simulink model "TST_InjCrv_PoI2"  (R2016b)
settings: Solver=FixedStepDiscrete  StartTime=0.0  StopTime=simTime  FixedStep=sampleTime  RelTol=1e-3
values from neighbouring files (symbols this model uses):
  testCase = 1    [initTST_InjCrv_PoI2_001.m]    (also in initTST_InjCrv_PoI2_002.m = 2)
libraries: simulink x6
settings Model: Creator=WF305  LastModifiedBy=WF305
settings DebuggingCC: SignalRangeChecking=error

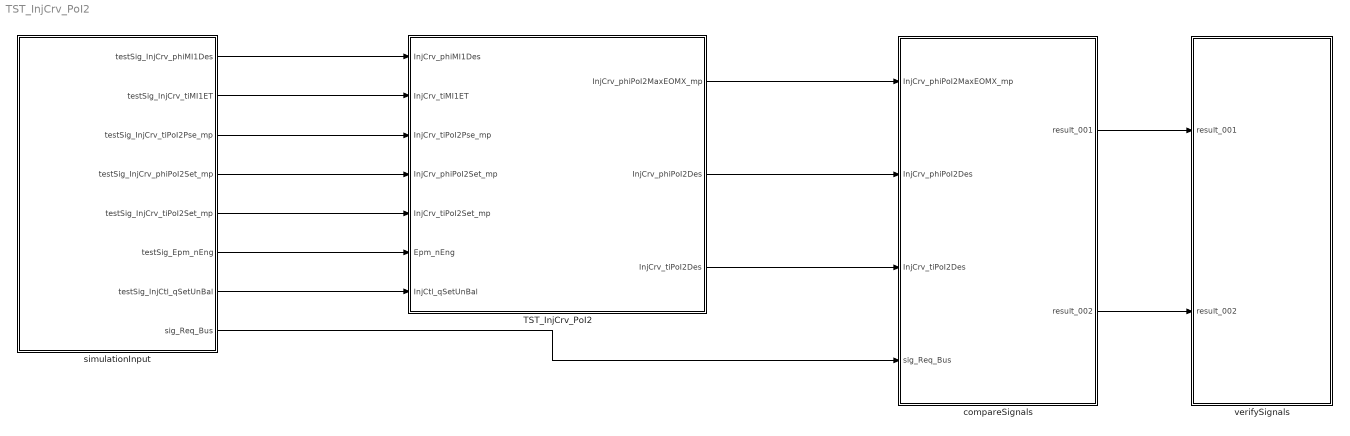
== system TST_InjCrv_PoI2 ==
  TST_InjCrv_PoI2 : Subsystem
  compareSignals : Subsystem
  simulationInput : Subsystem
  verifySignals : Subsystem
  wires:
  simulationInput/1(testSig_InjCrv_phiMI1Des) -> TST_InjCrv_PoI2/1(InjCrv_phiMI1Des)
  simulationInput/2(testSig_InjCrv_tiMI1ET) -> TST_InjCrv_PoI2/2(InjCrv_tiMI1ET)
  simulationInput/3(testSig_InjCrv_tiPoI2Pse_mp) -> TST_InjCrv_PoI2/3(InjCrv_tiPoI2Pse_mp)
  simulationInput/4(testSig_InjCrv_phiPoI2Set_mp) -> TST_InjCrv_PoI2/4(InjCrv_phiPoI2Set_mp)
  simulationInput/5(testSig_InjCrv_tiPoI2Set_mp) -> TST_InjCrv_PoI2/5(InjCrv_tiPoI2Set_mp)
  simulationInput/6(testSig_Epm_nEng) -> TST_InjCrv_PoI2/6(Epm_nEng)
  simulationInput/7(testSig_InjCtl_qSetUnBal) -> TST_InjCrv_PoI2/7(InjCtl_qSetUnBal)
  TST_InjCrv_PoI2/1(InjCrv_phiPoI2MaxEOMX_mp) -> compareSignals/1(InjCrv_phiPoI2MaxEOMX_mp)
  TST_InjCrv_PoI2/2(InjCrv_phiPoI2Des) -> compareSignals/2(InjCrv_phiPoI2Des)
  TST_InjCrv_PoI2/3(InjCrv_tiPoI2Des) -> compareSignals/3(InjCrv_tiPoI2Des)
  simulationInput/8(sig_Req_Bus) -> compareSignals/4(sig_Req_Bus)
  compareSignals/1(result_001) -> verifySignals/1(result_001)
  compareSignals/2(result_002) -> verifySignals/2(result_002)

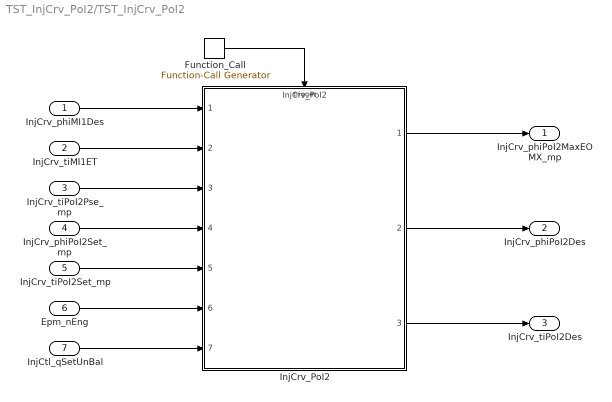
== system TST_InjCrv_PoI2/TST_InjCrv_PoI2 ==
  InjCrv_phiMI1Des : Inport
  InjCrv_tiMI1ET : Inport  Port=2
  InjCrv_tiPoI2Pse_mp : Inport  Port=3
  InjCrv_phiPoI2Set_mp : Inport  Port=4
  InjCrv_tiPoI2Set_mp : Inport  Port=5
  Epm_nEng : Inport  Port=6
  InjCtl_qSetUnBal : Inport  Port=7
  Function_Call : simulink/Ports & Subsystems/Function-Call Generator  sample_time=sampleTime  numberOfIterations=1
  InjCrv_PoI2 : ModelReference  ModelNameDialog=InjCrv_PoI2  ModelReferenceVersion=1.22  TriggerPortName=function  TriggerPortTriggerType=function-call  TriggerPortStatesWhenEnabling=held
  InjCrv_phiPoI2MaxEOMX_mp : Outport
  InjCrv_phiPoI2Des : Outport  Port=2
  InjCrv_tiPoI2Des : Outport  Port=3
  wires:
  Function_Call/1 -> InjCrv_PoI2/Trigger
  InjCrv_phiMI1Des/1 -> InjCrv_PoI2/1
  InjCrv_tiMI1ET/1 -> InjCrv_PoI2/2
  InjCrv_tiPoI2Pse_mp/1 -> InjCrv_PoI2/3
  InjCrv_phiPoI2Set_mp/1 -> InjCrv_PoI2/4
  InjCrv_tiPoI2Set_mp/1 -> InjCrv_PoI2/5
  Epm_nEng/1 -> InjCrv_PoI2/6
  InjCtl_qSetUnBal/1 -> InjCrv_PoI2/7
  InjCrv_PoI2/1 -> InjCrv_phiPoI2MaxEOMX_mp/1
  InjCrv_PoI2/2 -> InjCrv_phiPoI2Des/1
  InjCrv_PoI2/3 -> InjCrv_tiPoI2Des/1

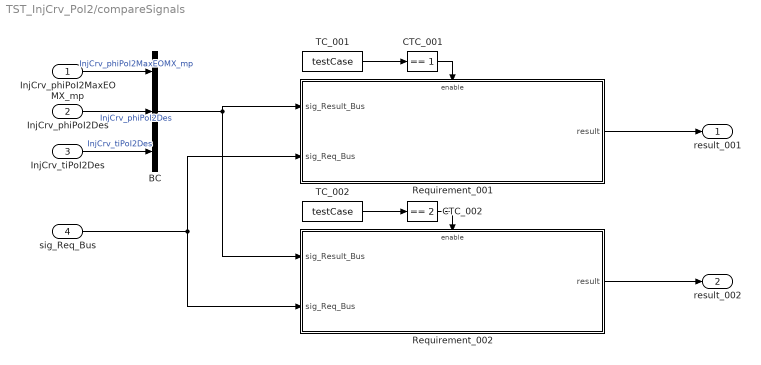
== system TST_InjCrv_PoI2/compareSignals ==
  InjCrv_phiPoI2MaxEOMX_mp : Inport
  InjCrv_phiPoI2Des : Inport  Port=2
  InjCrv_tiPoI2Des : Inport  Port=3
  sig_Req_Bus : Inport  Port=4
  BC : BusCreator  Inputs=3
  CTC_001 : simulink/Logic and Bit Operations/Compare To Constant  relop===  const=1  OutDataTypeStr=boolean
  CTC_002 : simulink/Logic and Bit Operations/Compare To Constant  relop===  const=2  OutDataTypeStr=boolean
  Requirement_001 : Subsystem
  Requirement_002 : Subsystem
  TC_001 : Constant  Value=testCase
  TC_002 : Constant  Value=testCase
  result_001 : Outport
  result_002 : Outport  Port=2
  wires:
  InjCrv_phiPoI2MaxEOMX_mp/1 -> BC/1  "InjCrv_phiPoI2MaxEOMX_mp"
  InjCrv_phiPoI2Des/1 -> BC/2  "InjCrv_phiPoI2Des"
  InjCrv_tiPoI2Des/1 -> BC/3  "InjCrv_tiPoI2Des"
  TC_001/1 -> CTC_001/1
  CTC_001/1 -> Requirement_001/Enable
  sig_Req_Bus/1 -> Requirement_001/2(sig_Req_Bus), Requirement_002/2(sig_Req_Bus)
  BC/1 -> Requirement_001/1(sig_Result_Bus), Requirement_002/1(sig_Result_Bus)
  Requirement_001/1(result) -> result_001/1
  TC_002/1 -> CTC_002/1
  CTC_002/1 -> Requirement_002/Enable
  Requirement_002/1(result) -> result_002/1

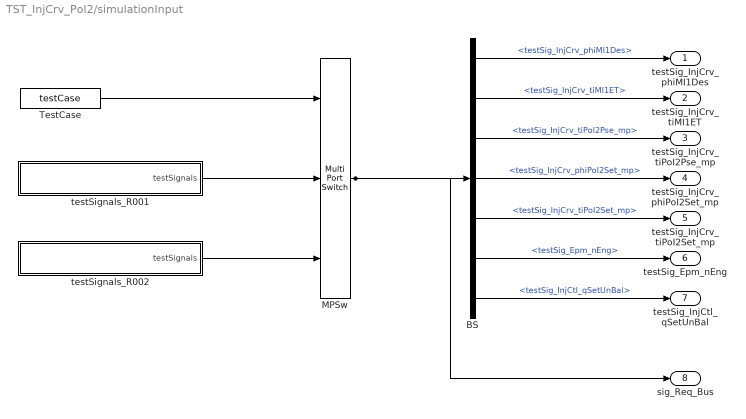
== system TST_InjCrv_PoI2/simulationInput ==
  BS : BusSelector  OutputSignals=testSig_InjCrv_phiMI1Des,testSig_InjCrv_tiMI1ET,testSig_InjCrv_tiPoI2Pse_mp,testSig_InjCrv_phiPoI2Set_mp,testSig_InjCrv_tiPoI2Set_mp,testSig_Epm_nEng,testSig_InjCtl_qSetUnBal
  MPSw : MultiPortSwitch  Inputs=2  SaturateOnIntegerOverflow=on  InputSameDT=on
  TestCase : Constant  Value=testCase
  testSignals_R001 : Subsystem
  testSignals_R002 : Subsystem
  testSig_InjCrv_phiMI1Des : Outport
  testSig_InjCrv_tiMI1ET : Outport  Port=2
  testSig_InjCrv_tiPoI2Pse_mp : Outport  Port=3
  testSig_InjCrv_phiPoI2Set_mp : Outport  Port=4
  testSig_InjCrv_tiPoI2Set_mp : Outport  Port=5
  testSig_Epm_nEng : Outport  Port=6
  testSig_InjCtl_qSetUnBal : Outport  Port=7
  sig_Req_Bus : Outport  Port=8
  wires:
  BS/1 -> testSig_InjCrv_phiMI1Des/1  "<testSig_InjCrv_phiMI1Des>"
  BS/2 -> testSig_InjCrv_tiMI1ET/1  "<testSig_InjCrv_tiMI1ET>"
  BS/3 -> testSig_InjCrv_tiPoI2Pse_mp/1  "<testSig_InjCrv_tiPoI2Pse_mp>"
  BS/4 -> testSig_InjCrv_phiPoI2Set_mp/1  "<testSig_InjCrv_phiPoI2Set_mp>"
  BS/5 -> testSig_InjCrv_tiPoI2Set_mp/1  "<testSig_InjCrv_tiPoI2Set_mp>"
  BS/6 -> testSig_Epm_nEng/1  "<testSig_Epm_nEng>"
  BS/7 -> testSig_InjCtl_qSetUnBal/1  "<testSig_InjCtl_qSetUnBal>"
  MPSw/1 -> BS/1, sig_Req_Bus/1
  TestCase/1 -> MPSw/1
  testSignals_R001/1(testSignals) -> MPSw/2
  testSignals_R002/1(testSignals) -> MPSw/3

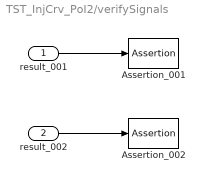
== system TST_InjCrv_PoI2/verifySignals ==
  result_001 : Inport
  result_002 : Inport  Port=2
  Assertion_001 : Assertion  Enabled=off
  Assertion_002 : Assertion  Enabled=off
  wires:
  result_001/1 -> Assertion_001/1
  result_002/1 -> Assertion_002/1

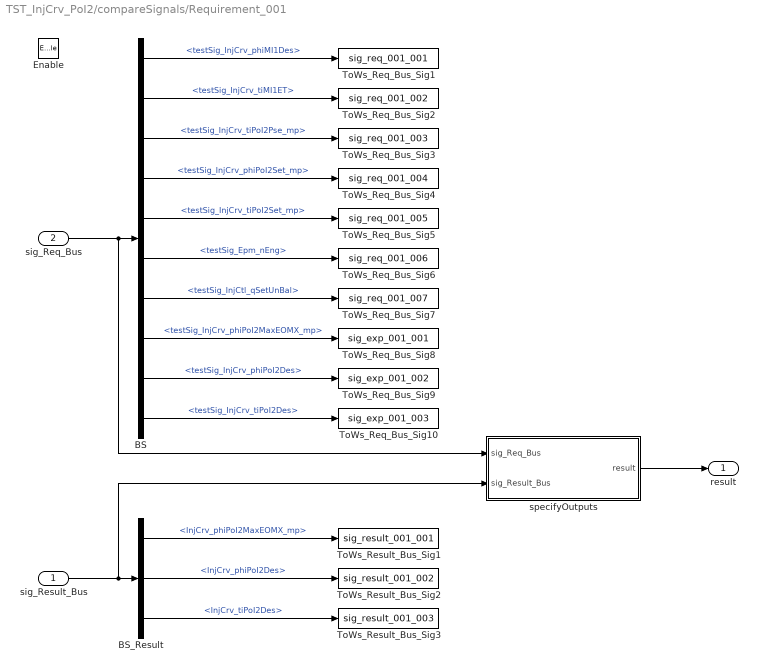
== system TST_InjCrv_PoI2/compareSignals/Requirement_001 ==
  sig_Result_Bus : Inport
  sig_Req_Bus : Inport  Port=2
  Enable : EnablePort
  BS : BusSelector  OutputSignals=testSig_InjCrv_phiMI1Des,testSig_InjCrv_tiMI1ET,testSig_InjCrv_tiPoI2Pse_mp,testSig_InjCrv_phiPoI2Set_mp,testSig_InjCrv_tiPoI2Set_mp,testSig_Epm_nEng,testSig_InjCtl_qSetUnBal,testSig_InjCrv_phiPoI2MaxEOMX_mp,testSig_InjCrv_phiPoI2Des,testSig_InjCrv_tiPoI2Des
  BS_Result : BusSelector  OutputSignals=InjCrv_phiPoI2MaxEOMX_mp,InjCrv_phiPoI2Des,InjCrv_tiPoI2Des
  ToWs_Req_Bus_Sig1 : ToWorkspace  VariableName=sig_req_001_001  SaveFormat=Structure With Time
  ToWs_Req_Bus_Sig10 : ToWorkspace  VariableName=sig_exp_001_003  SaveFormat=Structure With Time
  ToWs_Req_Bus_Sig2 : ToWorkspace  VariableName=sig_req_001_002  SaveFormat=Structure With Time
  ToWs_Req_Bus_Sig3 : ToWorkspace  VariableName=sig_req_001_003  SaveFormat=Structure With Time
  ToWs_Req_Bus_Sig4 : ToWorkspace  VariableName=sig_req_001_004  SaveFormat=Structure With Time
  ToWs_Req_Bus_Sig5 : ToWorkspace  VariableName=sig_req_001_005  SaveFormat=Structure With Time
  ToWs_Req_Bus_Sig6 : ToWorkspace  VariableName=sig_req_001_006  SaveFormat=Structure With Time
  ToWs_Req_Bus_Sig7 : ToWorkspace  VariableName=sig_req_001_007  SaveFormat=Structure With Time
  ToWs_Req_Bus_Sig8 : ToWorkspace  VariableName=sig_exp_001_001  SaveFormat=Structure With Time
  ToWs_Req_Bus_Sig9 : ToWorkspace  VariableName=sig_exp_001_002  SaveFormat=Structure With Time
  ToWs_Result_Bus_Sig1 : ToWorkspace  VariableName=sig_result_001_001  SaveFormat=Structure With Time
  ToWs_Result_Bus_Sig2 : ToWorkspace  VariableName=sig_result_001_002  SaveFormat=Structure With Time
  ToWs_Result_Bus_Sig3 : ToWorkspace  VariableName=sig_result_001_003  SaveFormat=Structure With Time
  specifyOutputs : Subsystem
  result : Outport
  wires:
  sig_Req_Bus/1 -> BS/1, specifyOutputs/1(sig_Req_Bus)
  BS/1 -> ToWs_Req_Bus_Sig1/1  "<testSig_InjCrv_phiMI1Des>"
  BS/2 -> ToWs_Req_Bus_Sig2/1  "<testSig_InjCrv_tiMI1ET>"
  BS/3 -> ToWs_Req_Bus_Sig3/1  "<testSig_InjCrv_tiPoI2Pse_mp>"
  BS/4 -> ToWs_Req_Bus_Sig4/1  "<testSig_InjCrv_phiPoI2Set_mp>"
  BS/5 -> ToWs_Req_Bus_Sig5/1  "<testSig_InjCrv_tiPoI2Set_mp>"
  BS/6 -> ToWs_Req_Bus_Sig6/1  "<testSig_Epm_nEng>"
  BS/7 -> ToWs_Req_Bus_Sig7/1  "<testSig_InjCtl_qSetUnBal>"
  BS/8 -> ToWs_Req_Bus_Sig8/1  "<testSig_InjCrv_phiPoI2MaxEOMX_mp>"
  BS/9 -> ToWs_Req_Bus_Sig9/1  "<testSig_InjCrv_phiPoI2Des>"
  BS/10 -> ToWs_Req_Bus_Sig10/1  "<testSig_InjCrv_tiPoI2Des>"
  sig_Result_Bus/1 -> BS_Result/1, specifyOutputs/2(sig_Result_Bus)
  BS_Result/1 -> ToWs_Result_Bus_Sig1/1  "<InjCrv_phiPoI2MaxEOMX_mp>"
  BS_Result/2 -> ToWs_Result_Bus_Sig2/1  "<InjCrv_phiPoI2Des>"
  BS_Result/3 -> ToWs_Result_Bus_Sig3/1  "<InjCrv_tiPoI2Des>"
  specifyOutputs/1(result) -> result/1

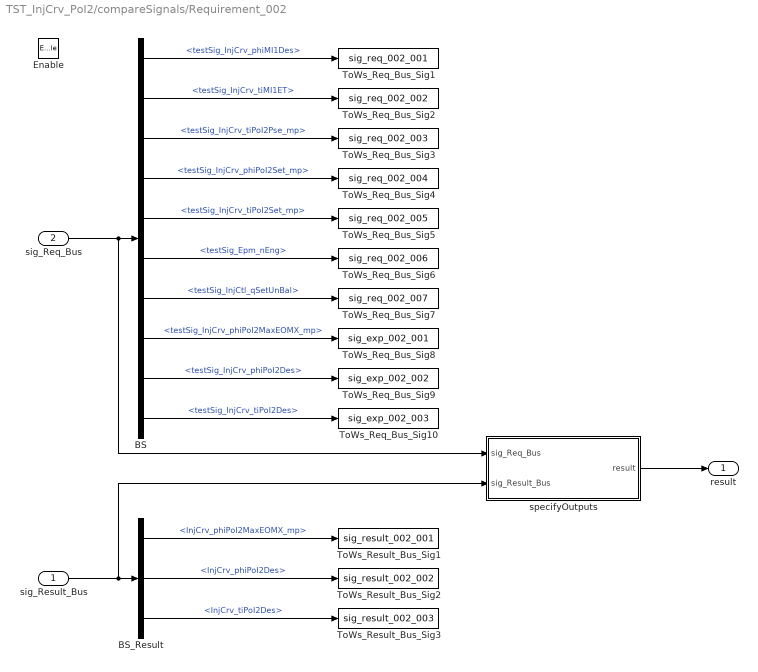
== system TST_InjCrv_PoI2/compareSignals/Requirement_002 ==
  sig_Result_Bus : Inport
  sig_Req_Bus : Inport  Port=2
  Enable : EnablePort
  BS : BusSelector  OutputSignals=testSig_InjCrv_phiMI1Des,testSig_InjCrv_tiMI1ET,testSig_InjCrv_tiPoI2Pse_mp,testSig_InjCrv_phiPoI2Set_mp,testSig_InjCrv_tiPoI2Set_mp,testSig_Epm_nEng,testSig_InjCtl_qSetUnBal,testSig_InjCrv_phiPoI2MaxEOMX_mp,testSig_InjCrv_phiPoI2Des,testSig_InjCrv_tiPoI2Des
  BS_Result : BusSelector  OutputSignals=InjCrv_phiPoI2MaxEOMX_mp,InjCrv_phiPoI2Des,InjCrv_tiPoI2Des
  ToWs_Req_Bus_Sig1 : ToWorkspace  VariableName=sig_req_002_001  SaveFormat=Structure With Time
  ToWs_Req_Bus_Sig10 : ToWorkspace  VariableName=sig_exp_002_003  SaveFormat=Structure With Time
  ToWs_Req_Bus_Sig2 : ToWorkspace  VariableName=sig_req_002_002  SaveFormat=Structure With Time
  ToWs_Req_Bus_Sig3 : ToWorkspace  VariableName=sig_req_002_003  SaveFormat=Structure With Time
  ToWs_Req_Bus_Sig4 : ToWorkspace  VariableName=sig_req_002_004  SaveFormat=Structure With Time
  ToWs_Req_Bus_Sig5 : ToWorkspace  VariableName=sig_req_002_005  SaveFormat=Structure With Time
  ToWs_Req_Bus_Sig6 : ToWorkspace  VariableName=sig_req_002_006  SaveFormat=Structure With Time
  ToWs_Req_Bus_Sig7 : ToWorkspace  VariableName=sig_req_002_007  SaveFormat=Structure With Time
  ToWs_Req_Bus_Sig8 : ToWorkspace  VariableName=sig_exp_002_001  SaveFormat=Structure With Time
  ToWs_Req_Bus_Sig9 : ToWorkspace  VariableName=sig_exp_002_002  SaveFormat=Structure With Time
  ToWs_Result_Bus_Sig1 : ToWorkspace  VariableName=sig_result_002_001  SaveFormat=Structure With Time
  ToWs_Result_Bus_Sig2 : ToWorkspace  VariableName=sig_result_002_002  SaveFormat=Structure With Time
  ToWs_Result_Bus_Sig3 : ToWorkspace  VariableName=sig_result_002_003  SaveFormat=Structure With Time
  specifyOutputs : Subsystem
  result : Outport
  wires:
  sig_Req_Bus/1 -> BS/1, specifyOutputs/1(sig_Req_Bus)
  BS/1 -> ToWs_Req_Bus_Sig1/1  "<testSig_InjCrv_phiMI1Des>"
  BS/2 -> ToWs_Req_Bus_Sig2/1  "<testSig_InjCrv_tiMI1ET>"
  BS/3 -> ToWs_Req_Bus_Sig3/1  "<testSig_InjCrv_tiPoI2Pse_mp>"
  BS/4 -> ToWs_Req_Bus_Sig4/1  "<testSig_InjCrv_phiPoI2Set_mp>"
  BS/5 -> ToWs_Req_Bus_Sig5/1  "<testSig_InjCrv_tiPoI2Set_mp>"
  BS/6 -> ToWs_Req_Bus_Sig6/1  "<testSig_Epm_nEng>"
  BS/7 -> ToWs_Req_Bus_Sig7/1  "<testSig_InjCtl_qSetUnBal>"
  BS/8 -> ToWs_Req_Bus_Sig8/1  "<testSig_InjCrv_phiPoI2MaxEOMX_mp>"
  BS/9 -> ToWs_Req_Bus_Sig9/1  "<testSig_InjCrv_phiPoI2Des>"
  BS/10 -> ToWs_Req_Bus_Sig10/1  "<testSig_InjCrv_tiPoI2Des>"
  sig_Result_Bus/1 -> BS_Result/1, specifyOutputs/2(sig_Result_Bus)
  BS_Result/1 -> ToWs_Result_Bus_Sig1/1  "<InjCrv_phiPoI2MaxEOMX_mp>"
  BS_Result/2 -> ToWs_Result_Bus_Sig2/1  "<InjCrv_phiPoI2Des>"
  BS_Result/3 -> ToWs_Result_Bus_Sig3/1  "<InjCrv_tiPoI2Des>"
  specifyOutputs/1(result) -> result/1

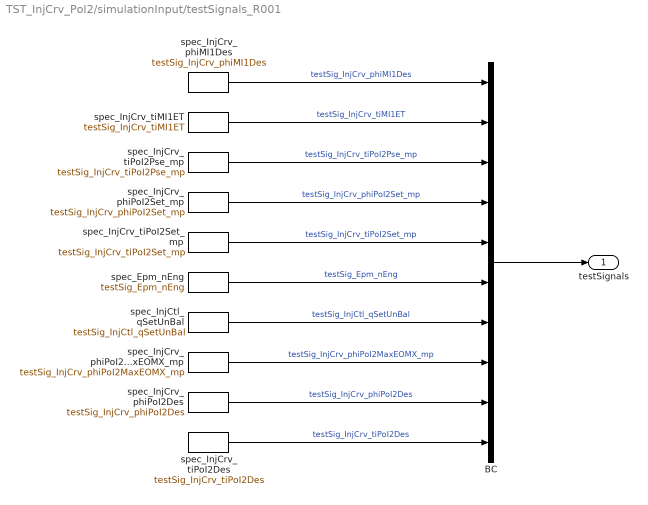
== system TST_InjCrv_PoI2/simulationInput/testSignals_R001 ==
  BC : BusCreator  Inputs=10
  spec_Epm_nEng : FromWorkspace  VariableName=testSig_Epm_nEng  Interpolate=off  OutputAfterFinalValue=Holding final value
  spec_InjCrv_phiMI1Des : FromWorkspace  VariableName=testSig_InjCrv_phiMI1Des  Interpolate=off  OutputAfterFinalValue=Holding final value
  spec_InjCrv_phiPoI2Des : FromWorkspace  VariableName=testSig_InjCrv_phiPoI2Des  Interpolate=off  OutputAfterFinalValue=Holding final value
  spec_InjCrv_phiPoI2MaxEOMX_mp : FromWorkspace  VariableName=testSig_InjCrv_phiPoI2MaxEOMX_mp  Interpolate=off  OutputAfterFinalValue=Holding final value
  spec_InjCrv_phiPoI2Set_mp : FromWorkspace  VariableName=testSig_InjCrv_phiPoI2Set_mp  Interpolate=off  OutputAfterFinalValue=Holding final value
  spec_InjCrv_tiMI1ET : FromWorkspace  VariableName=testSig_InjCrv_tiMI1ET  Interpolate=off  OutputAfterFinalValue=Holding final value
  spec_InjCrv_tiPoI2Des : FromWorkspace  VariableName=testSig_InjCrv_tiPoI2Des  Interpolate=off  OutputAfterFinalValue=Holding final value
  spec_InjCrv_tiPoI2Pse_mp : FromWorkspace  VariableName=testSig_InjCrv_tiPoI2Pse_mp  Interpolate=off  OutputAfterFinalValue=Holding final value
  spec_InjCrv_tiPoI2Set_mp : FromWorkspace  VariableName=testSig_InjCrv_tiPoI2Set_mp  Interpolate=off  OutputAfterFinalValue=Holding final value
  spec_InjCtl_qSetUnBal : FromWorkspace  VariableName=testSig_InjCtl_qSetUnBal  Interpolate=off  OutputAfterFinalValue=Holding final value
  testSignals : Outport
  wires:
  BC/1 -> testSignals/1
  spec_InjCrv_phiMI1Des/1 -> BC/1  "testSig_InjCrv_phiMI1Des"
  spec_InjCrv_tiMI1ET/1 -> BC/2  "testSig_InjCrv_tiMI1ET"
  spec_InjCrv_tiPoI2Pse_mp/1 -> BC/3  "testSig_InjCrv_tiPoI2Pse_mp"
  spec_InjCrv_phiPoI2Set_mp/1 -> BC/4  "testSig_InjCrv_phiPoI2Set_mp"
  spec_InjCrv_tiPoI2Set_mp/1 -> BC/5  "testSig_InjCrv_tiPoI2Set_mp"
  spec_Epm_nEng/1 -> BC/6  "testSig_Epm_nEng"
  spec_InjCtl_qSetUnBal/1 -> BC/7  "testSig_InjCtl_qSetUnBal"
  spec_InjCrv_phiPoI2MaxEOMX_mp/1 -> BC/8  "testSig_InjCrv_phiPoI2MaxEOMX_mp"
  spec_InjCrv_phiPoI2Des/1 -> BC/9  "testSig_InjCrv_phiPoI2Des"
  spec_InjCrv_tiPoI2Des/1 -> BC/10  "testSig_InjCrv_tiPoI2Des"

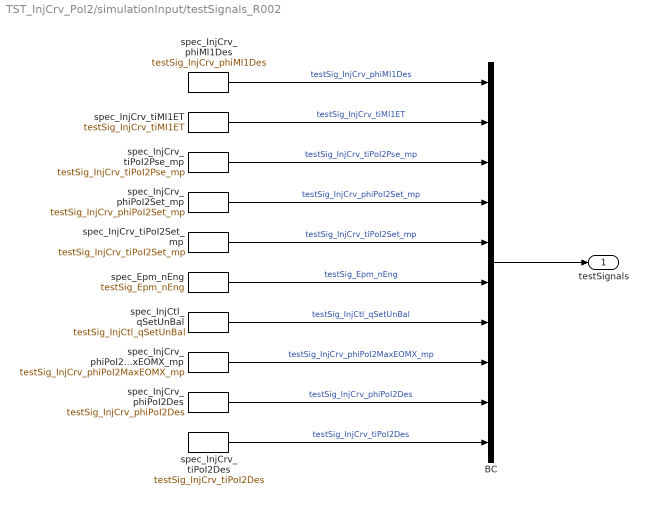
== system TST_InjCrv_PoI2/simulationInput/testSignals_R002 ==
  BC : BusCreator  Inputs=10
  spec_Epm_nEng : FromWorkspace  VariableName=testSig_Epm_nEng  Interpolate=off  OutputAfterFinalValue=Holding final value
  spec_InjCrv_phiMI1Des : FromWorkspace  VariableName=testSig_InjCrv_phiMI1Des  Interpolate=off  OutputAfterFinalValue=Holding final value
  spec_InjCrv_phiPoI2Des : FromWorkspace  VariableName=testSig_InjCrv_phiPoI2Des  Interpolate=off  OutputAfterFinalValue=Holding final value
  spec_InjCrv_phiPoI2MaxEOMX_mp : FromWorkspace  VariableName=testSig_InjCrv_phiPoI2MaxEOMX_mp  Interpolate=off  OutputAfterFinalValue=Holding final value
  spec_InjCrv_phiPoI2Set_mp : FromWorkspace  VariableName=testSig_InjCrv_phiPoI2Set_mp  Interpolate=off  OutputAfterFinalValue=Holding final value
  spec_InjCrv_tiMI1ET : FromWorkspace  VariableName=testSig_InjCrv_tiMI1ET  Interpolate=off  OutputAfterFinalValue=Holding final value
  spec_InjCrv_tiPoI2Des : FromWorkspace  VariableName=testSig_InjCrv_tiPoI2Des  Interpolate=off  OutputAfterFinalValue=Holding final value
  spec_InjCrv_tiPoI2Pse_mp : FromWorkspace  VariableName=testSig_InjCrv_tiPoI2Pse_mp  Interpolate=off  OutputAfterFinalValue=Holding final value
  spec_InjCrv_tiPoI2Set_mp : FromWorkspace  VariableName=testSig_InjCrv_tiPoI2Set_mp  Interpolate=off  OutputAfterFinalValue=Holding final value
  spec_InjCtl_qSetUnBal : FromWorkspace  VariableName=testSig_InjCtl_qSetUnBal  Interpolate=off  OutputAfterFinalValue=Holding final value
  testSignals : Outport
  wires:
  BC/1 -> testSignals/1
  spec_InjCrv_phiMI1Des/1 -> BC/1  "testSig_InjCrv_phiMI1Des"
  spec_InjCrv_tiMI1ET/1 -> BC/2  "testSig_InjCrv_tiMI1ET"
  spec_InjCrv_tiPoI2Pse_mp/1 -> BC/3  "testSig_InjCrv_tiPoI2Pse_mp"
  spec_InjCrv_phiPoI2Set_mp/1 -> BC/4  "testSig_InjCrv_phiPoI2Set_mp"
  spec_InjCrv_tiPoI2Set_mp/1 -> BC/5  "testSig_InjCrv_tiPoI2Set_mp"
  spec_Epm_nEng/1 -> BC/6  "testSig_Epm_nEng"
  spec_InjCtl_qSetUnBal/1 -> BC/7  "testSig_InjCtl_qSetUnBal"
  spec_InjCrv_phiPoI2MaxEOMX_mp/1 -> BC/8  "testSig_InjCrv_phiPoI2MaxEOMX_mp"
  spec_InjCrv_phiPoI2Des/1 -> BC/9  "testSig_InjCrv_phiPoI2Des"
  spec_InjCrv_tiPoI2Des/1 -> BC/10  "testSig_InjCrv_tiPoI2Des"

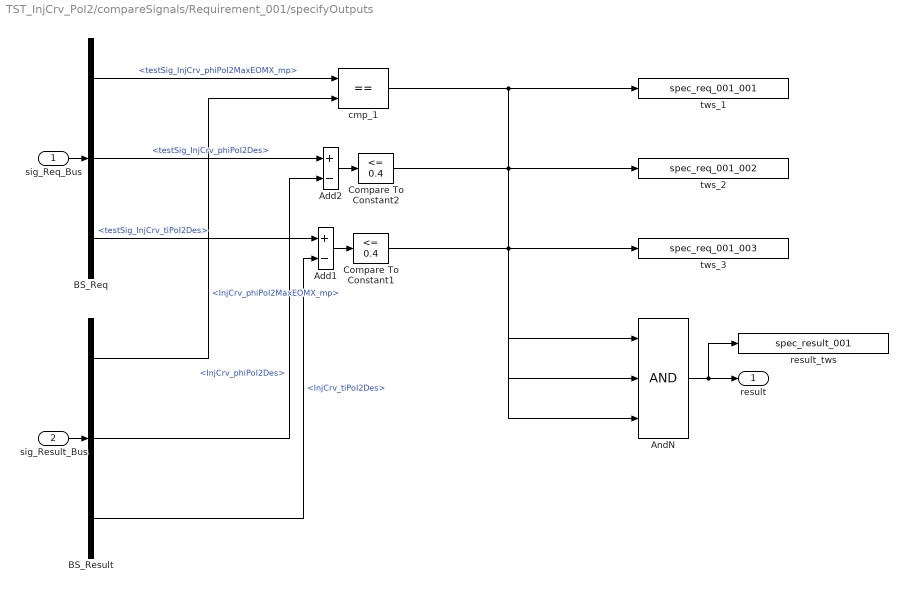
== system TST_InjCrv_PoI2/compareSignals/Requirement_001/specifyOutputs ==
  sig_Req_Bus : Inport
  sig_Result_Bus : Inport  Port=2
  Add1 : Sum  Inputs=+-
  Add2 : Sum  Inputs=+-
  AndN : Logic  Inputs=3
  BS_Req : BusSelector  OutputSignals=testSig_InjCrv_phiPoI2MaxEOMX_mp,testSig_InjCrv_phiPoI2Des,testSig_InjCrv_tiPoI2Des
  BS_Result : BusSelector  OutputSignals=InjCrv_phiPoI2MaxEOMX_mp,InjCrv_phiPoI2Des,InjCrv_tiPoI2Des
  Compare To Constant1 : simulink/Logic and Bit Operations/Compare To Constant  relop=<=  const=0.4  OutDataTypeStr=boolean
  Compare To Constant2 : simulink/Logic and Bit Operations/Compare To Constant  relop=<=  const=0.4  OutDataTypeStr=boolean
  cmp_1 : RelationalOperator  Operator===  RndMeth=Nearest  InputSameDT=on
  result_tws : ToWorkspace  VariableName=spec_result_001
  tws_1 : ToWorkspace  VariableName=spec_req_001_001
  tws_2 : ToWorkspace  VariableName=spec_req_001_002
  tws_3 : ToWorkspace  VariableName=spec_req_001_003
  result : Outport
  wires:
  sig_Req_Bus/1 -> BS_Req/1
  sig_Result_Bus/1 -> BS_Result/1
  AndN/1 -> result/1, result_tws/1
  BS_Req/1 -> cmp_1/1  "<testSig_InjCrv_phiPoI2MaxEOMX_mp>"
  BS_Result/1 -> cmp_1/2  "<InjCrv_phiPoI2MaxEOMX_mp>"
  cmp_1/1 -> tws_1/1, AndN/1
  BS_Req/2 -> Add2/1  "<testSig_InjCrv_phiPoI2Des>"
  BS_Result/2 -> Add2/2  "<InjCrv_phiPoI2Des>"
  Compare To Constant2/1 -> tws_2/1, AndN/2
  BS_Req/3 -> Add1/1  "<testSig_InjCrv_tiPoI2Des>"
  BS_Result/3 -> Add1/2  "<InjCrv_tiPoI2Des>"
  Compare To Constant1/1 -> tws_3/1, AndN/3
  Add1/1 -> Compare To Constant1/1
  Add2/1 -> Compare To Constant2/1

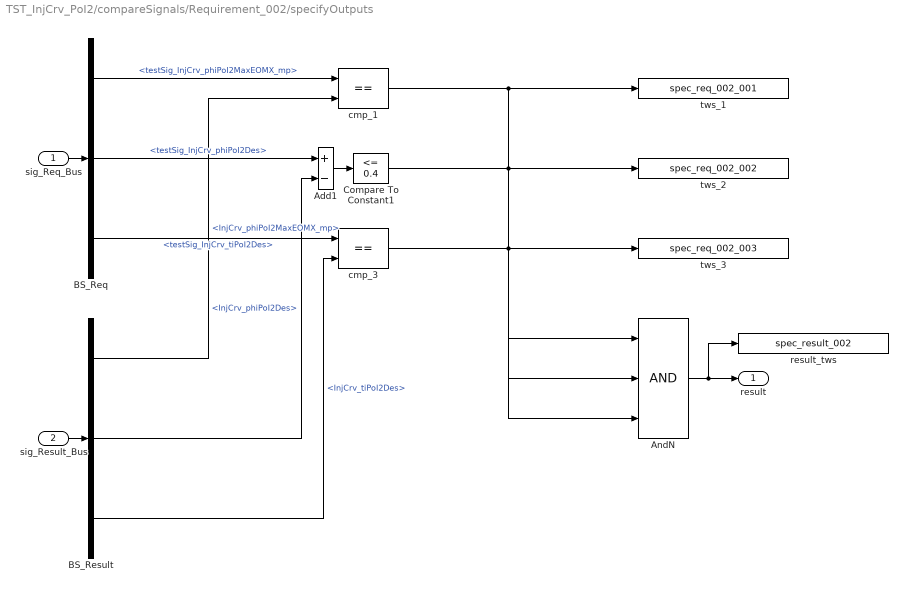
== system TST_InjCrv_PoI2/compareSignals/Requirement_002/specifyOutputs ==
  sig_Req_Bus : Inport
  sig_Result_Bus : Inport  Port=2
  Add1 : Sum  Inputs=+-
  AndN : Logic  Inputs=3
  BS_Req : BusSelector  OutputSignals=testSig_InjCrv_phiPoI2MaxEOMX_mp,testSig_InjCrv_phiPoI2Des,testSig_InjCrv_tiPoI2Des
  BS_Result : BusSelector  OutputSignals=InjCrv_phiPoI2MaxEOMX_mp,InjCrv_phiPoI2Des,InjCrv_tiPoI2Des
  Compare To Constant1 : simulink/Logic and Bit Operations/Compare To Constant  relop=<=  const=0.4  OutDataTypeStr=boolean
  cmp_1 : RelationalOperator  Operator===  RndMeth=Nearest  InputSameDT=on
  cmp_3 : RelationalOperator  Operator===  RndMeth=Nearest  InputSameDT=on
  result_tws : ToWorkspace  VariableName=spec_result_002
  tws_1 : ToWorkspace  VariableName=spec_req_002_001
  tws_2 : ToWorkspace  VariableName=spec_req_002_002
  tws_3 : ToWorkspace  VariableName=spec_req_002_003
  result : Outport
  wires:
  sig_Req_Bus/1 -> BS_Req/1
  sig_Result_Bus/1 -> BS_Result/1
  AndN/1 -> result/1, result_tws/1
  BS_Req/1 -> cmp_1/1  "<testSig_InjCrv_phiPoI2MaxEOMX_mp>"
  BS_Result/1 -> cmp_1/2  "<InjCrv_phiPoI2MaxEOMX_mp>"
  cmp_1/1 -> tws_1/1, AndN/1
  BS_Req/2 -> Add1/1  "<testSig_InjCrv_phiPoI2Des>"
  BS_Result/2 -> Add1/2  "<InjCrv_phiPoI2Des>"
  Compare To Constant1/1 -> tws_2/1, AndN/2
  BS_Req/3 -> cmp_3/1  "<testSig_InjCrv_tiPoI2Des>"
  BS_Result/3 -> cmp_3/2  "<InjCrv_tiPoI2Des>"
  cmp_3/1 -> tws_3/1, AndN/3
  Add1/1 -> Compare To Constant1/1
